simulink model "FA"  (R2024b)
settings: Solver=VariableStepAuto  StartTime=0.0  StopTime=10.0  RelTol=1e-3
settings Model: Creator=Shreesha Kumar  LastModifiedBy=Shreesha Kumar

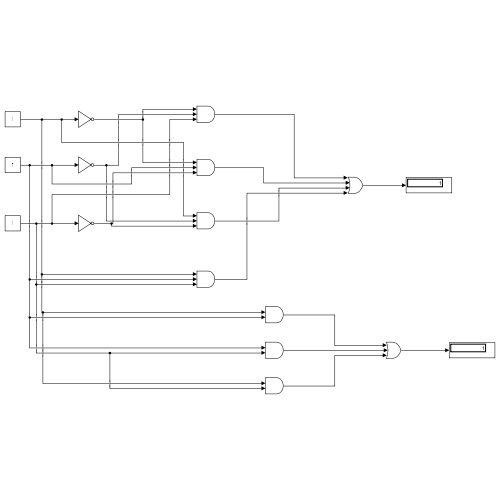
[thumbnail: Simulink's stored preview of the top-level diagram]
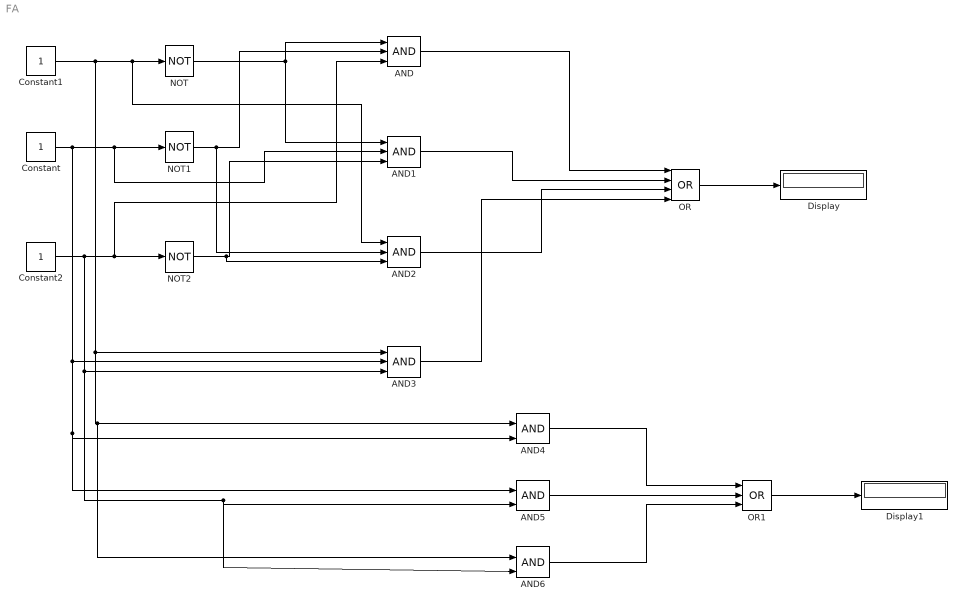
== system FA ==
  AND{,1..3} (4 alike) : Logic  Inputs=3  IconShape=distinctive  AllPortsSameDT=off  OutDataTypeStr=boolean
  AND4 : Logic  IconShape=distinctive  AllPortsSameDT=off  OutDataTypeStr=boolean
  AND5 : Logic  IconShape=distinctive  AllPortsSameDT=off  OutDataTypeStr=boolean
  AND6 : Logic  IconShape=distinctive  AllPortsSameDT=off  OutDataTypeStr=boolean
  Constant : Constant
  Constant1 : Constant
  Constant2 : Constant
  Display : Display
  Display1 : Display
  NOT : Logic  Operator=NOT  IconShape=distinctive  AllPortsSameDT=off  OutDataTypeStr=boolean
  NOT1 : Logic  Operator=NOT  IconShape=distinctive  AllPortsSameDT=off  OutDataTypeStr=boolean
  NOT2 : Logic  Operator=NOT  IconShape=distinctive  AllPortsSameDT=off  OutDataTypeStr=boolean
  OR : Logic  Operator=OR  Inputs=4  IconShape=distinctive  AllPortsSameDT=off  OutDataTypeStr=boolean
  OR1 : Logic  Operator=OR  Inputs=3  IconShape=distinctive  AllPortsSameDT=off  OutDataTypeStr=boolean
  wires:
  Constant1/1 -> AND6/1, AND4/1, AND3/1, AND2/1, NOT/1
  Constant/1 -> AND5/1, AND4/2, AND3/2, AND1/2, NOT1/1
  Constant2/1 -> AND6/2, AND5/2, AND3/3, AND/3, NOT2/1
  NOT/1 -> AND/1, AND1/1
  NOT1/1 -> AND2/2, AND/2
  NOT2/1 -> AND2/3, AND1/3
  AND6/1 -> OR1/3
  AND5/1 -> OR1/2
  AND4/1 -> OR1/1
  AND/1 -> OR/1
  AND1/1 -> OR/2
  AND2/1 -> OR/3
  OR/1 -> Display/1
  OR1/1 -> Display1/1
  AND3/1 -> OR/4
